simulink model "modelo_blocos"  (R2017a)
settings: Solver=VariableStepAuto  StartTime=0.0  StopTime=10  MaxStep=0.0001  RelTol=1e-6
values from neighbouring files (symbols this model uses):
  a = -subs(y_lin, [y yd u], [0 1 0])    [linearization.m]    (also in preConfig.m = 0.97)
  b = -subs(y_lin, [y yd u], [1 0 0])    [linearization.m]    (also in preConfig.m = 6.4)
  g = 9.8    [preConfig.m]
  m = 0.12    [preConfig.m]
  N = 4    [preConfig.m]
libraries: simulink x1
settings Model: Creator=Herculano  LastModifiedBy=Herculano

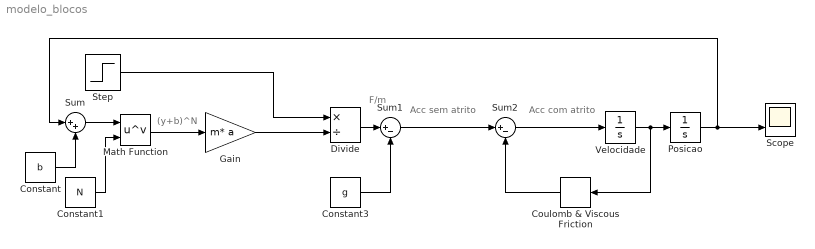
== system modelo_blocos ==
  note: Acc com atrito
  note: Acc sem atrito
  note: F/m
  note: (y+b)^N
  Constant : Constant  Value=b
  Constant1 : Constant  Value=N
  Constant3 : Constant  Value=g
  Coulomb & Viscous Friction : simulink/Discontinuities/Coulomb & Viscous Friction  offset=0  gain=15/12
      settings: SourceProductName=Simulink
  Divide : Product  Inputs=*/
  Gain : Gain  Gain=m* a
  Math Function : Math  Operator=pow  SaturateOnIntegerOverflow=on
  Posicao : Integrator
  Scope : Scope  NumInputPorts=2
  Step : Step  Time=0  After=20000  SampleTime=0
  Sum : Sum  Inputs=|++
  Sum1 : Sum  Inputs=|+-
  Sum2 : Sum  Inputs=|+-
  "Velocidade " : Integrator
  wires:
  Divide/1 -> Sum1/1
  Constant1/1 -> Math Function/2
  Math Function/1 -> Gain/1
  Constant3/1 -> Sum1/2
  Sum/1 -> Math Function/1
  Constant/1 -> Sum/2
  Posicao/1 -> Scope/2, Sum/1
  Step/1 -> Divide/1
  "Velocidade "/1 -> Posicao/1, Coulomb & Viscous Friction/1
  Gain/1 -> Divide/2
  Coulomb & Viscous Friction/1 -> Sum2/2
  Sum1/1 -> Sum2/1
  Sum2/1 -> "Velocidade "/1
